simulink model "Pre_9_1"  (R2014a)
settings: Solver=ode45  StartTime=0.0  StopTime=10000  RelTol=1e-3
libraries: hdlsllib x1
settings Model: Creator=Shiyu  LastModifiedBy=Shiyu

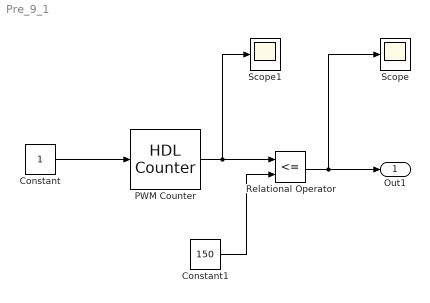
== system Pre_9_1 ==
  Constant : Constant  OutDataTypeStr=boolean
  Constant1 : Constant  Value=150  OutDataTypeStr=uint8  SampleTime=1
  PWM Counter : hdlsllib/HDL Operations/HDL Counter  CountType=Count limited  CountInit=0  CountStep=1  CountMax=2000  CountFromType=Initial value  CountFrom=0  CountResetPort=off  CountLoadPort=off  CountEnbPort=on  CountDirPort=off  CountDataType=Unsigned  CountWordLen=16  CountFracLen=0  CountSampTime=1
  Relational Operator : RelationalOperator  Operator=<=  OutDataTypeStr=boolean  SampleTime=1
  Scope : Scope
  Scope1 : Scope
  Out1 : Outport  OutDataTypeStr=boolean
  wires:
  PWM Counter/1 -> Relational Operator/1, Scope1/1
  Relational Operator/1 -> Scope/1, Out1/1
  Constant1/1 -> Relational Operator/2
  Constant/1 -> PWM Counter/1
